simulink model "PID_controller"  (R2020a)
settings: Solver=VariableStepAuto  StartTime=0.0  StopTime=10  RelTol=1e-3
undefined symbols (not defined in the file or in its folder): Kd, Ki, Kp, N
settings Model: DataDictionary=Motorpos.sldd  Creator=USER  LastModifiedBy=USER
settings DataIOCC: SaveOutput=off  SaveTime=off

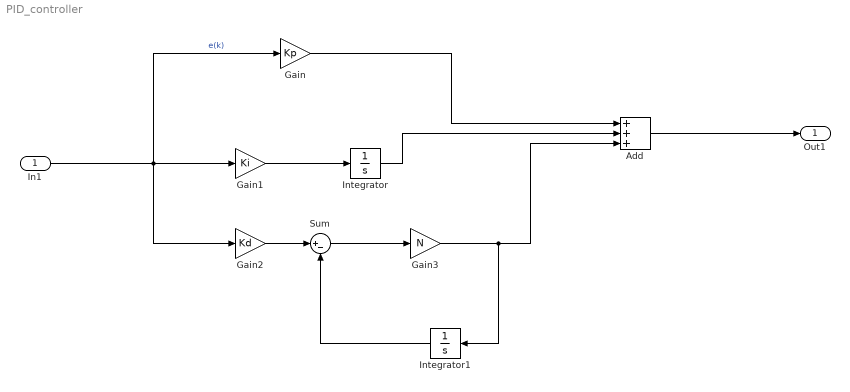
== system PID_controller ==
  In1 : Inport  OutDataTypeStr=double  PortDimensions=1  SampleTime=0
  Add : Sum  Inputs=+++
  Gain : Gain  Gain=Kp
  Gain1 : Gain  Gain=Ki
  Gain2 : Gain  Gain=Kd
  Gain3 : Gain  Gain=N
  Integrator : Integrator
  Integrator1 : Integrator
  Sum : Sum  Inputs=|+-
  Out1 : Outport  OutDataTypeStr=double  PortDimensions=1  SampleTime=0
  wires:
  Gain/1 -> Add/1
  In1/1 -> Gain/1, Gain1/1, Gain2/1  "e(k)"
  Gain1/1 -> Integrator/1
  Gain2/1 -> Sum/1
  Integrator/1 -> Add/2
  Add/1 -> Out1/1
  Integrator1/1 -> Sum/2
  Gain3/1 -> Add/3, Integrator1/1
  Sum/1 -> Gain3/1
